simulink model "ex_DLModel"  (R2023b)
settings: Solver=FixedStepAuto  StartTime=0.0  StopTime=inf  FixedStep=0.05  RelTol=1e-3
libraries: nvidiaAVlib x2, deeplib x1
settings Model: Creator=The MathWorks, Inc.  LastModifiedBy=TechsourceDeviceEnro
settings SolverCC: AlgebraicLoopSolver=TrustRegion
settings OptimizationCC: EnhancedBackFolding=on  PassReuseOutputArgsAs=Individual arguments  ZeroExternalMemoryAtStartup=off  ZeroInternalMemoryAtStartup=off  InitFltsAndDblsToZero=on  MaxStackSize=64  OptimizeBlockOrder=speed  DifferentSizesBufferReuse=on  OptimizationCustomize=off  EfficientTunableParamExpr=on
settings DebuggingCC: ParameterTunabilityLossMsg=error  UnconnectedInputMsg=warning  UnconnectedOutputMsg=warning  UnconnectedLineMsg=warning
settings HardwareCC: ProdBitPerLong=64  ProdLargestAtomicInteger=LongLong  ProdLargestAtomicFloat=Double  ProdLongLongMode=on  ProdHWDeviceType=ARM Compatible->ARM 64-bit (LP64)  TargetLongLongMode=on
settings ModelReferenceCC: EnableRefExpFcnMdlSchedulingChecks=on
settings RTWCC: Description=Embedded Coder  SystemTargetFile=ert.tlc  HardwareBoard=NVIDIA Jetson  TLCOptions="-aInlineSetEventsForThisBaseRateFcn=TLC_FALSE -aSuppressMultiTaskScheduler=TLC_FALSE  -aRateBasedStepFcn=0"  TemplateMakefile=ert_default_tmf  Toolchain=NVCC for NVIDIA Embedded Processors  TargetLang=C++  GenerateGPUCode=CUDA  DLTargetLibrary=cudnn  DLArmComputeVersion=19.05
settings CodeAppCC: ForceParamTrailComments=on  IgnoreCustomStorageClasses=off  OperatorAnnotations=on  SimulinkDataObjDesc=on  SFDataObjDesc=on  InsertBlockDesc=on
settings ERTTargetCC: CodeInterfacePackaging=C++ class  SupportVariableSizeSignals=on  RootIOFormat=Structure reference

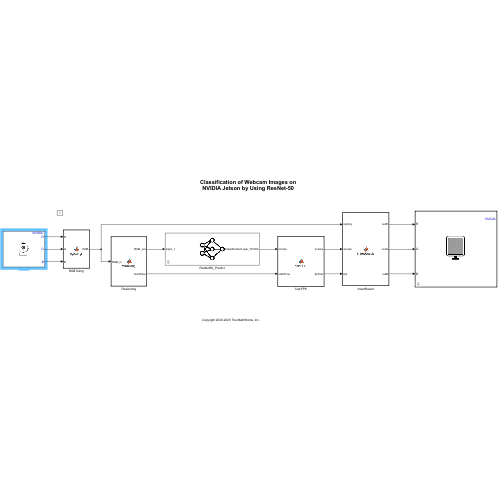
[thumbnail: Simulink's stored preview of the top-level diagram]
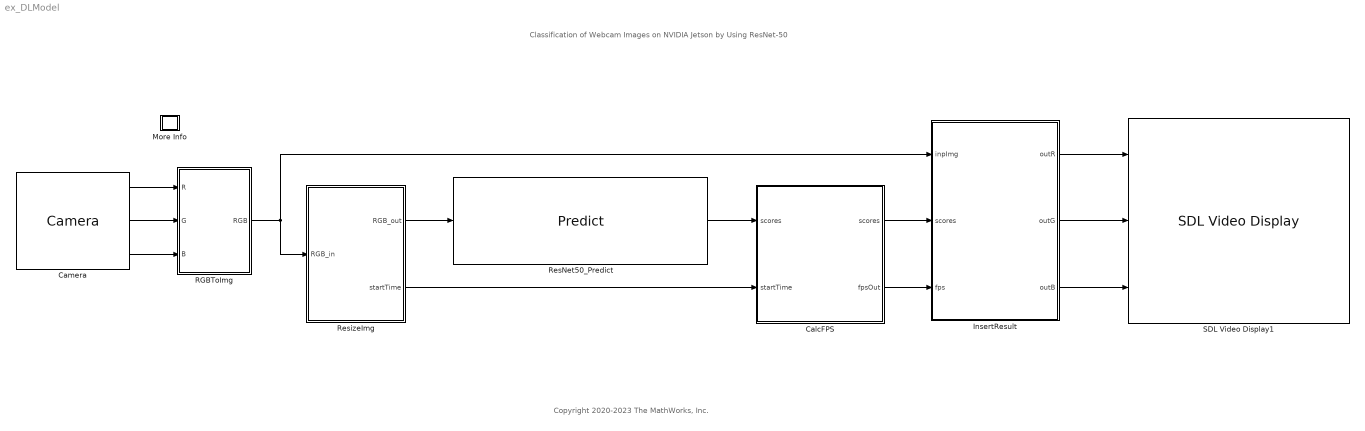
== system ex_DLModel ==
  note: Copyright 2020-2023 The MathWorks, Inc.
  note: Classification of Webcam Images on NVIDIA Jetson by Using ResNet-50
  CalcFPS : MATLAB Function  TreatAsAtomicUnit=on
  Camera : nvidiaAVlib/Camera  CameraName=UVC Camera (046d:0825)  ImageSize=[320,240]  SampleTime=0.2  SimulateUsing=Code generation
  InsertResult : MATLAB Function  TreatAsAtomicUnit=on
  More Info : Subsystem
      settings: OpenFcn=showExample('stats/PredictClassLabelsUsingMATLABFunctionBlockExample')
      mask Display: disp('?')
  RGBToImg : MATLAB Function  TreatAsAtomicUnit=on
  ResNet50_Predict : deeplib/Predict  Network=Network from MATLAB function  NetworkFunction=resnet50  NetworkFilePath=[]  MiniBatchSize=128  InputDataFormats={ '', '' }  Predictions=on  Activations={}  ForceInterpretedSim=off  EnableDLNetwork=off
  ResizeImg : MATLAB Function  TreatAsAtomicUnit=on
  SDL Video Display1 : nvidiaAVlib/SDL Video Display  pixelFormat=RGB  pixelOrder=Planar  rowMajor=on  blockPlatform=NVIDIA
  wires:
  ResizeImg/1(RGB_out) -> ResNet50_Predict/1
  InsertResult/3(outB) -> SDL Video Display1/3
  InsertResult/2(outG) -> SDL Video Display1/2
  Camera/3 -> RGBToImg/3(B)
  CalcFPS/2(fpsOut) -> InsertResult/3(fps)
  Camera/2 -> RGBToImg/2(G)
  ResNet50_Predict/1 -> CalcFPS/1("scores ")
  RGBToImg/1(RGB) -> InsertResult/1(inpImg), ResizeImg/1(RGB_in)
  Camera/1 -> RGBToImg/1(R)
  ResizeImg/2(startTime) -> CalcFPS/2(startTime)
  CalcFPS/1(scores) -> InsertResult/2(scores)
  InsertResult/1(outR) -> SDL Video Display1/1

== system ex_DLModel/More Info ==

== matlab function ex_DLModel/RGBToImg ==
  data: R input; RGB output; G input; B input
function RGB  = rgb2Img(R,G,B)
RGB = coder.nullcopy(uint8(zeros(size(R,1),size(R,2),3)));
RGB(:,:,1) = R;
RGB(:,:,2) = G;
RGB(:,:,3) = B;
end

== matlab function ex_DLModel/ResizeImg ==
  data: RGB_in input; RGB_out output; startTime output
function [RGB_out, startTime] = resizeImg(RGB_in)
RGB_out = imresize(RGB_in,[224,224]);
currentTime = datetime;
startTime = [currentTime.Year currentTime.Month currentTime.Day currentTime.Hour ...
    currentTime.Minute currentTime.Second];

== matlab function ex_DLModel/InsertResult ==
  data: inpImg input; outR output; scores input; outG output; outB output; fps input
function [outR,outG,outB] = insertResult(inpImg, scores, fps)

[scores,index] = sort(scores,'descend');

%% Insert prediction with scores in the image

%Pad Image
outImg = padarray(inpImg,[0,200],0,'pre');

index5 = index(1:5);
synsetData = coder.load('synsetWords.mat');
synsetData = synsetData.synsetArray;

outImg = insertText(outImg, [10 80],['FPS : ' sprintf('%0.2f',fps) ], 'AnchorPoint','LeftBottom');

for i=1:5
   str = strtrim(synsetData(index5(i),:));
   outImg = insertText(outImg, [10 50+30*(i+1)],[str ': ' sprintf('%0.2f',scores(i)*100) '%'], 'AnchorPoint','LeftBottom');
end

outR = outImg(:,:,1)';
outG = outImg(:,:,2)';
outB = outImg(:,:,3)';

== matlab function ex_DLModel/CalcFPS ==
  data: scores input; startTime input; scores output; fpsOut output
function [scores,fpsOut] = calcFPS(scores, startTime)
finishTime = datetime;

diffTime = seconds(finishTime-datetime(startTime));
persistent count;
if isempty(count)
    count = 0;
end
persistent fps;
if isempty(fps)
    fps = 0;
end
fps = (count*fps + 1*(1/diffTime))/(count+1);

count = count + 1;
fpsOut = fps;
